simulink model "Tirocinio4Parte2"  (R2025b)
settings: Solver=VariableStepAuto  StartTime=0.0  StopTime=150  RelTol=1e-6  AbsTol=1e-6
values from neighbouring files (symbols this model uses):
  A2 = [0 0 1 0 ; 0 0 0 1; -k2/m1_2 k2/m1_2 -c2/m1_2 c2/m1_2; k2/m2_2 -k2/m2_2 c2/m2_2 -c2/m2_2]    [Tirocinio3.m]    (also in Tirocinio4.m = [0 0 1 0;0 0 0 1;-k/m1 k/m1 -c/m1 c/m1;k/m2 -k/m2 c/m2 -c/m2)
  B2 = [0 0 1/m1_2 0]'    [Tirocinio3.m]    (also in Tirocinio4.m = [0 0 1/m1 0]')
  C2 = [1 0 0 0]    [Tirocinio3.m]    (also in Tirocinio4.m)
  M2 = [0 0 0 1/m2_2]'    [Tirocinio3.m]    (also in Tirocinio4.m = 2)
  OM = 1    [Tirocinio4.m]
  phase = 1    [Tirocinio4.m]
undefined symbols (not defined in the file or in its folder): A_comp_sin, A_reale, B_comp_sin, B_reale, C_comp_sin, C_reale
settings Model: Creator=sarab  LastModifiedBy=Davide

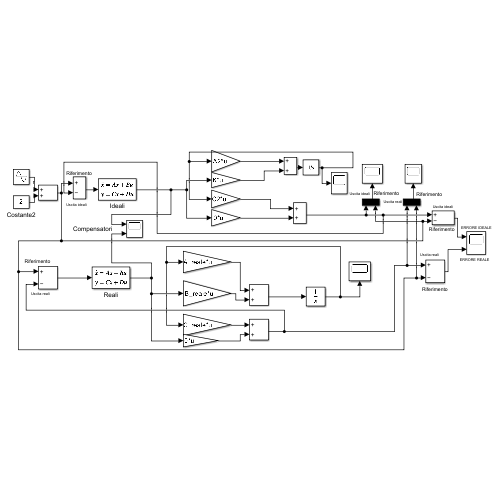
[thumbnail: Simulink's stored preview of the top-level diagram]
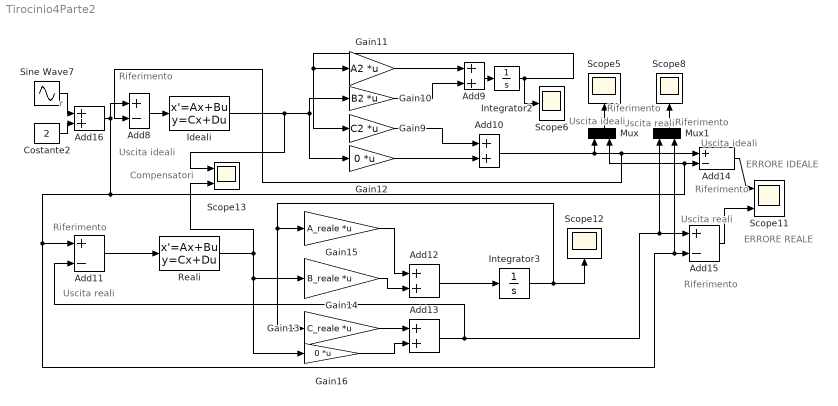
== system Tirocinio4Parte2 ==
  note: Compensatori
  note: Uscita reali
  note: Riferimento
  note: ERRORE REALE
  note: ERRORE IDEALE
  note: Riferimento
  note: Uscita ideali
  note: Riferimento
  note: Uscita reali
  note: Uscita reali
  note: Riferimento
  note: Uscita ideali
  note: Riferimento
  note: Uscita ideali
  note: Riferimento
  Add{9..10,12..13,16} (5 alike) : Sum
  Add{8,11,14..15} (4 alike) : Sum  Inputs=+-
  Costante2 : Constant  Value=2
  Gain10 : Gain  Gain=B2  Multiplication=Matrix(K*u)
  Gain11 : Gain  Gain=A2  Multiplication=Matrix(K*u)
  Gain12 : Gain  Gain=0  Multiplication=Matrix(K*u)
  Gain13 : Gain  Gain=C_reale  Multiplication=Matrix(K*u)
  Gain14 : Gain  Gain=B_reale  Multiplication=Matrix(K*u)
  Gain15 : Gain  Gain=A_reale  Multiplication=Matrix(K*u)
  Gain16 : Gain  Gain=0  Multiplication=Matrix(K*u)
  Gain9 : Gain  Gain=C2  Multiplication=Matrix(K*u)
  Ideali : StateSpace  A=A_comp_sin  B=B_comp_sin  C=C_comp_sin  D=0  InitialCondition=0
  Integrator2 : Integrator  InitialCondition=[0 0 0 0]  AbsoluteTolerance=1
  Integrator3 : Integrator  InitialCondition=[0 0 0 0]  AbsoluteTolerance=1
  Mux : Mux  Inputs=2
  Mux1 : Mux  Inputs=2
  Reali : StateSpace  A=A_comp_sin  B=B_comp_sin  C=C_comp_sin  D=0  InitialCondition=0
  Scope11 : Scope  NumInputPorts=2
      settings: ActiveDisplayYMinimum=-8.5242862125973176  ActiveDisplayYMaximum=14.479257195028714  DataLoggingVariableName=ScopeData9
  Scope{5..6,8,12} (4 alike) : Scope
      Scope12 settings: ActiveDisplayYMinimum=-12.687303500895991  ActiveDisplayYMaximum=10.232879677114356  DataLoggingVariableName=ScopeData10
      Scope5 settings: ActiveDisplayYMinimum=-6.9333638746693156  ActiveDisplayYMaximum=6.4675925315806886  DataLoggingVariableName=ScopeData3
      Scope6 settings: ActiveDisplayYMinimum=-14.325358278823565  ActiveDisplayYMaximum=12.20761877262067  DataLoggingVariableName=ScopeData4
      Scope8 settings: ActiveDisplayYMinimum=-10.142916847630914  ActiveDisplayYMaximum=9.656399146763075  DataLoggingVariableName=ScopeData11
  Scope13 : Scope  NumInputPorts=2
      settings: ActiveDisplayYMinimum=-67.90692908180155  ActiveDisplayYMaximum=68.698302801796373  DataLoggingVariableName=ScopeData8
  Sine Wave7 : Sin  Amplitude=M2  Frequency=OM  Phase=phase  SampleTime=0
  wires:
  Add8/1 -> Ideali/1
  Ideali/1 -> Scope13/1, Gain12/1, Gain10/1
  Gain11/1 -> Add9/1
  Gain10/1 -> Add9/2
  Add9/1 -> Integrator2/1
  Integrator2/1 -> Gain9/1, Gain11/1, Scope6/1
  Gain9/1 -> Add10/1
  Gain12/1 -> Add10/2
  Add10/1 -> Add14/1, Add8/2, Mux/1
  Add11/1 -> Reali/1
  Reali/1 -> Gain16/1, Gain14/1, Scope13/2
  Gain15/1 -> Add12/1
  Gain14/1 -> Add12/2
  Add12/1 -> Integrator3/1
  Integrator3/1 -> Scope12/1, Gain15/1, Gain13/1
  Gain13/1 -> Add13/1
  Gain16/1 -> Add13/2
  Add13/1 -> Add15/1, Mux1/1, Add11/2
  Add14/1 -> Scope11/1
  Add15/1 -> Scope11/2
  Mux/1 -> Scope5/1
  Mux1/1 -> Scope8/1
  Sine Wave7/1 -> Add16/1  "r"
  Costante2/1 -> Add16/2
  Add16/1 -> Add14/2, Mux/2, Add11/1, Mux1/2, Add15/2, Add8/1
